simulink model "Day3_5_1"  (R2022b)
settings: Solver=FixedStepAuto  StartTime=0.0  StopTime=inf  FixedStep=0.01  RelTol=1e-3
values from neighbouring files (symbols this model uses):
  Ki = 1    [Day3_5.m]
  Kp = 1    [Day3_5.m]
settings Model: Creator=user  LastModifiedBy=user

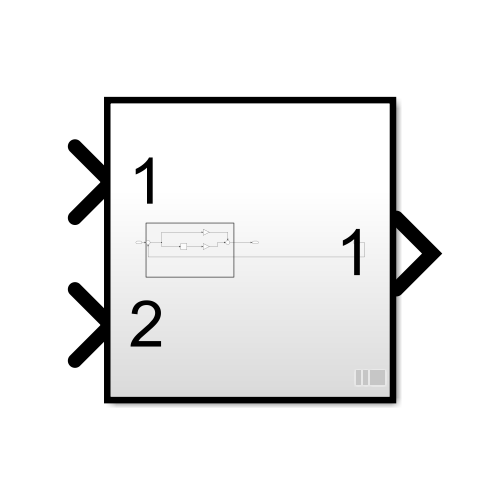
[thumbnail: Simulink's stored preview of the top-level diagram]
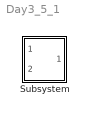
== system Day3_5_1 ==
  Subsystem : Subsystem  TreatAsAtomicUnit=on

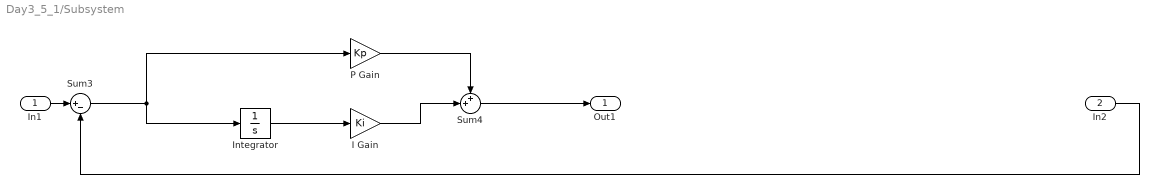
== system Day3_5_1/Subsystem ==
  In1 : Inport
  In2 : Inport  Port=2
  I Gain : Gain  Gain=Ki
  Integrator : Integrator
  P Gain : Gain  Gain=Kp
  Sum3 : Sum  Inputs=|+-
  Sum4 : Sum  Inputs=++|
  Out1 : Outport
  wires:
  Sum4/1 -> Out1/1
  In1/1 -> Sum3/1
  Integrator/1 -> I Gain/1
  P Gain/1 -> Sum4/1
  I Gain/1 -> Sum4/2
  Sum3/1 -> P Gain/1, Integrator/1
  In2/1 -> Sum3/2
